simulink model "lidar_webcam_im"  (Simulink 7.3)
settings: Solver=FixedStepDiscrete  StartTime=0.0  StopTime=inf  MaxStep=0.2  RelTol=1e-3
settings Model: Creator=gclayton  LastModifiedBy=wildcat
settings DebuggingCC: InheritedTsInSrcMsg=none
settings RTWCC: SystemTargetFile=rlnx.tlc  GenCodeOnly=on  TemplateMakefile=rlnx_ubuntu.tmf  Description=Linux Real-Time Target  ProcessScript=rlnx_make_rtw_hook
settings RTWCC: CustomInclude=|
  | /usr/local/include/opencv/
  | /usr/local/include/
settings CodeAppCC: GenerateComments=off  SimulinkBlockComments=off
settings STFCustomTargetCC: ModelReferenceCompliant=off  MatFileLogging=on  SystemTargetFile=rlnx.tlc
settings GRTTargetCC: ModelReferenceCompliant=off  ParMdlRefBuildCompliant=off  CompOptLevelCompliant=off
settings CustomProperty: DataType=string  Value=-lm -ldl /usr/local/lib/libopencv_highgui.so.2.4 /usr/local/lib/libopencv_core.so.2.4 /usr/local/lib/libopencv_imgproc.so.2.4 -lc_urg -lc_urg_connection -lc_urg_system -lphidget21
settings EnumStrPairs: String=PC

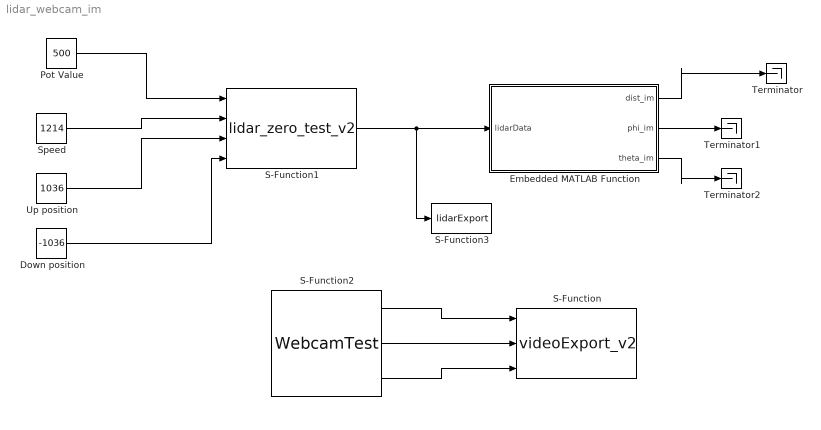
== system lidar_webcam_im ==
  Down position : Constant  Value=-1036  OutDataType=fixdt(1, 16)  OutScaling=2^0
  Embedded MATLAB Function : Stateflow chart
  Pot Value : Constant  Value=500  OutDataTypeMode=int32  OutDataType=fixdt(1, 16)  OutScaling=2^0  OutDataTypeStr=int32
  S-Function : S-Function  FunctionName=videoExport_v2  EnableBusSupport=off
  S-Function1 : S-Function  FunctionName=lidar_zero_test_v2  EnableBusSupport=off
  S-Function2 : S-Function  FunctionName=WebcamTest  EnableBusSupport=off
  S-Function3 : S-Function  FunctionName=lidarExport  EnableBusSupport=off
  Speed : Constant  Value=1214  OutDataType=fixdt(1, 16)  OutScaling=2^0
  Terminator : Terminator
  Terminator1 : Terminator
  Terminator2 : Terminator
  Up position : Constant  Value=1036  OutDataType=fixdt(1, 16)  OutScaling=2^0
  wires:
  S-Function1/1 -> S-Function3/1, Embedded MATLAB Function/1(lidarData)
  Speed/1 -> S-Function1/2
  Up position/1 -> S-Function1/3
  Down position/1 -> S-Function1/4
  S-Function2/3 -> S-Function/3
  S-Function2/2 -> S-Function/2
  S-Function2/1 -> S-Function/1
  Pot Value/1 -> S-Function1/1
  Embedded MATLAB Function/1(dist_im) -> Terminator/1
  Embedded MATLAB Function/2(phi_im) -> Terminator1/1
  Embedded MATLAB Function/3(theta_im) -> Terminator2/1

== matlab function Embedded MATLAB Function ==
  data: lidarData input double; dist_im output double; phi_im output double; theta_im output double
function [dist_im, phi_im, theta_im] = image_creator(lidarData)
%#eml

% Define variables based on gimbal system and scan pattern
ScanNum = 65;
DataLength = 1080*ScanNum;
h = 36.3;

% Define Data sizes
phim = zeros(1,DataLength);
thetam = zeros(1,DataLength);
distm = zeros(1,DataLength);
dist_im = zeros(ScanNum,600);
phi_im = zeros(ScanNum,600);
theta_im = zeros(ScanNum,600);


%Define phi_rad: angles corresponding to one lidar scan
l = 1:1080;
phi_rad = (-45 + 0.25*l)*pi/180;

% Repeat phim for number of scans
for i = 1:ScanNum
        
    for j = 1 : 1080
        phi_val = 1080*(i-1) + j;
        phim(1,phi_val) = phi_rad(1,j);
    end
end

% Theta changes from -45 to 45 degrees over the duration of the scan
theta_min = -45*pi/180;
theta_max = 45*pi/180;
theta_step = (theta_max - theta_min)/DataLength;
thetam = [theta_max : -theta_step : (theta_min+theta_step)];

% Distance matrix is directly from lidar data
distm = lidarData';


% Create images for distance, phi, and theta
for i2 = 1:ScanNum
    for j2 = 1:600
        dist_im(i2,j2) = distm(1, 240+j2 + 1080*(i2-1));
        phi_im(i2,j2) = phim(1, 240+j2 + 1080*(i2-1));
        theta_im(i2,j2) = thetam(1, 240+j2 + 1080*(i2-1));
    end
    
end
